simulink model "GotoGoal"  (R2017b)
settings: Solver=VariableStepAuto  StartTime=0.0  StopTime=time  RelTol=1e-3
values from neighbouring files (symbols this model uses):
  K = 0.1705+0.0007    (= 0.1712)    [CinematicaDirec.m]
  L = 25    [CinematicaDirec.m]
  R = 10    [CinematicaDirec.m]
  tau_1 = 0.0448+0.0019    (= 0.0467)    [CinematicaDirec.m]
  tau_2 = 0.6282+0.0018    (= 0.63)    [CinematicaDirec.m]
  x = zeros(1,tiempo)    [Controlador.m]
  y = zeros(1,tiempo)    [Controlador.m]
undefined symbols (not defined in the file or in its folder): magnitude
settings Model: Creator=nicolasfelipevergaraduran  LastModifiedBy=nicolasfelipevergaraduran

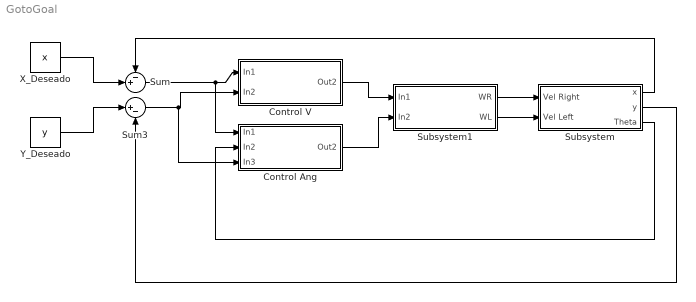
== system GotoGoal ==
  "Control Ang " : Subsystem
  Control V : Subsystem
  Subsystem : Subsystem
  Subsystem1 : Subsystem
  Sum : Sum  Inputs=-+|
  Sum3 : Sum  Inputs=|+-
  X_Deseado : Constant  Value=x
  "Y_Deseado " : Constant  Value=y
  wires:
  "Y_Deseado "/1 -> Sum3/1
  Subsystem/2(y) -> Sum3/2
  Sum/1 -> "Control Ang "/1(In1), Control V/1(In1)
  Subsystem/3(Theta) -> "Control Ang "/2(In2)
  Subsystem1/1(WR) -> Subsystem/1("Vel Right ")
  Subsystem/1(x) -> Sum/1
  X_Deseado/1 -> Sum/2
  Sum3/1 -> "Control Ang "/3(In3), Control V/2(In2)
  Subsystem1/2(WL) -> Subsystem/2("Vel Left ")
  "Control Ang "/1(Out2) -> Subsystem1/2(In2)
  Control V/1(Out2) -> Subsystem1/1(In1)

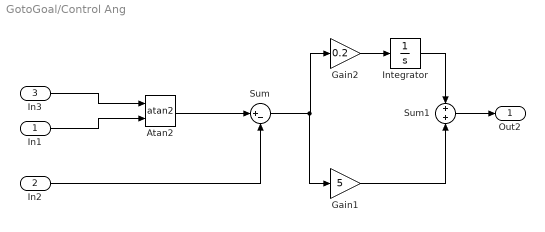
== system GotoGoal/Control Ang  ==
  In1 : Inport
  In2 : Inport  Port=2
  In3 : Inport  Port=3
  Atan2 : Trigonometry  Operator=atan2
  Gain1 : Gain  Gain=5
  Gain2 : Gain  Gain=0.2
  Integrator : Integrator
  Sum : Sum  Inputs=|+-
  Sum1 : Sum  Inputs=+|+
  Out2 : Outport
  wires:
  In2/1 -> Sum/2
  In1/1 -> Atan2/2
  In3/1 -> Atan2/1
  Gain2/1 -> Integrator/1
  Integrator/1 -> Sum1/1
  Gain1/1 -> Sum1/2
  Sum/1 -> Gain2/1, Gain1/1
  Atan2/1 -> Sum/1
  Sum1/1 -> Out2/1

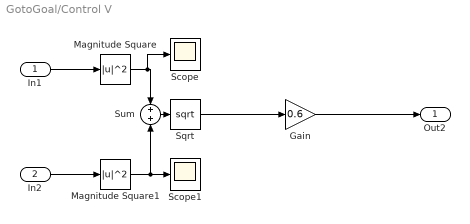
== system GotoGoal/Control V ==
  In1 : Inport
  In2 : Inport  Port=2
  Gain : Gain  Gain=0.6
  Magnitude Square : Math  Operator=magnitude^2  RndMeth=Zero  SaturateOnIntegerOverflow=on
  Magnitude Square1 : Math  Operator=magnitude^2  RndMeth=Zero  SaturateOnIntegerOverflow=on
  Scope : Scope
  Scope1 : Scope
  Sqrt : Sqrt  SaturateOnIntegerOverflow=on
  Sum : Sum  Inputs=+|+
  Out2 : Outport
  wires:
  Sqrt/1 -> Gain/1
  In2/1 -> Magnitude Square1/1
  Sum/1 -> Sqrt/1
  Magnitude Square/1 -> Scope/1, Sum/1
  Magnitude Square1/1 -> Scope1/1, Sum/2
  In1/1 -> Magnitude Square/1
  Gain/1 -> Out2/1

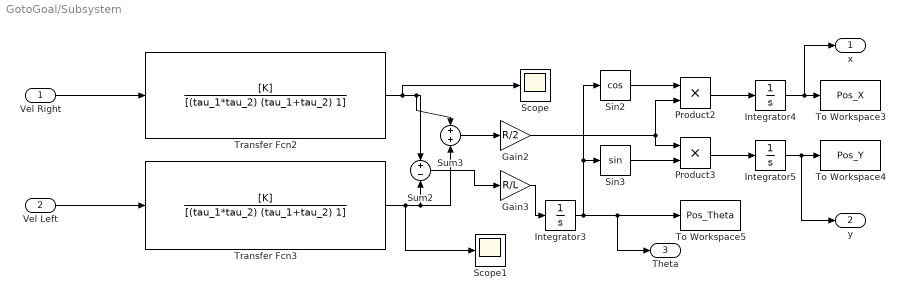
== system GotoGoal/Subsystem ==
  "Vel Right " : Inport
  "Vel Left " : Inport  Port=2
  Gain2 : Gain  Gain=R/2
  Gain3 : Gain  Gain=R/L
  Integrator3 : Integrator
  Integrator4 : Integrator
  Integrator5 : Integrator
  Product2 : Product
  Product3 : Product
  Scope : Scope
  Scope1 : Scope
  Sin2 : Trigonometry  Operator=cos
  Sin3 : Trigonometry
  Sum2 : Sum  Inputs=+|-
  Sum3 : Sum  Inputs=+|+
  To Workspace3 : ToWorkspace  VariableName=Pos_X  SaveFormat=Timeseries  SampleTime=-1
  To Workspace4 : ToWorkspace  VariableName=Pos_Y  SaveFormat=Timeseries  SampleTime=-1
  To Workspace5 : ToWorkspace  VariableName=Pos_Theta  SaveFormat=Timeseries  SampleTime=-1
  Transfer Fcn2 : TransferFcn  Numerator=[K]  Denominator=[(tau_1*tau_2) (tau_1+tau_2) 1]
  Transfer Fcn3 : TransferFcn  Numerator=[K]  Denominator=[(tau_1*tau_2) (tau_1+tau_2) 1]
  x : Outport
  y : Outport  Port=2
  Theta : Outport  Port=3
  wires:
  Transfer Fcn2/1 -> Scope/1, Sum3/1, Sum2/1
  Sin3/1 -> Product3/2
  Integrator3/1 -> Theta/1, To Workspace5/1, Sin3/1, Sin2/1
  Product2/1 -> Integrator4/1
  Sin2/1 -> Product2/1
  Sum3/1 -> Gain2/1
  Sum2/1 -> Gain3/1
  Gain2/1 -> Product3/1, Product2/2
  Gain3/1 -> Integrator3/1
  Product3/1 -> Integrator5/1
  Integrator4/1 -> x/1, To Workspace3/1
  Integrator5/1 -> y/1, To Workspace4/1
  Transfer Fcn3/1 -> Scope1/1, Sum3/2, Sum2/2
  "Vel Right "/1 -> Transfer Fcn2/1
  "Vel Left "/1 -> Transfer Fcn3/1

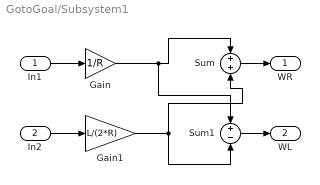
== system GotoGoal/Subsystem1 ==
  In1 : Inport
  In2 : Inport  Port=2
  Gain : Gain  Gain=1/R
  Gain1 : Gain  Gain=L/(2*R)
  Sum : Sum  Inputs=+|+
  Sum1 : Sum  Inputs=+|-
  WR : Outport
  WL : Outport  Port=2
  wires:
  Sum/1 -> WR/1
  Sum1/1 -> WL/1
  In1/1 -> Gain/1
  In2/1 -> Gain1/1
  Gain/1 -> Sum1/1, Sum/1
  Gain1/1 -> Sum1/2, Sum/2
